simulink model "threephasethyristor"  (R2016a)
settings: Solver=VariableStepAuto  StartTime=0.0  StopTime=1  RelTol=1e-3
libraries: powerlib x21, powerlib_meascontrol x3, dspstat3 x1
settings Model: Creator=hakan  LastModifiedBy=hakan

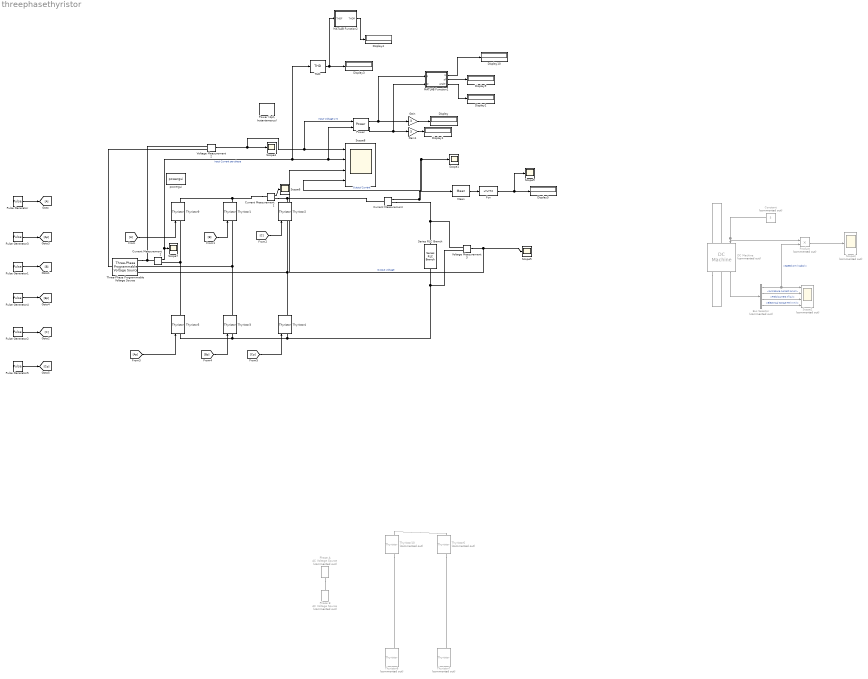
== system threephasethyristor ==
  Bus Selector : BusSelector  Commented=on  OutputSignals=Speed wm (rad/s),Armature current ia (A),Field current if (A),Electrical torque Te (n m)
  Constant : Constant  Commented=on  Value=5
  Current Measurement : powerlib/Measurements/Current Measurement  PhasorSimulation=off  OutputType=Complex  PSBequivalent=0
  Current Measurement1 : powerlib/Measurements/Current Measurement  PhasorSimulation=off  OutputType=Complex  PSBequivalent=0
  Current Measurement2 : powerlib/Measurements/Current Measurement  PhasorSimulation=off  OutputType=Complex  PSBequivalent=0
  DC Machine : powerlib/Machines/DC Machine  Commented=on  PresetModel=No  MechanicalLoad=Torque TL  FieldType=Wound  ShowDetailedParameters=on  MeasurementBus=off  RLa="[ 28  0.0133]"  RLf="[8260  6.4]"  Laf=1.5  MachineConstant=Torque constant (N.m/A)  Ke=1.8  Kt=1.8  J=1  Bm=0  Tf=0  w0=1  Ifinit=1  TsPowergui=0  TsBlock=-1
  Display{,1..5,9..10} (8 alike) : Display
  Fcn : Fcn  Expr=u*u*72
  Gain : Gain  Gain=3
  Gain1 : Gain  Gain=3
  MATLAB Function1 : MATLAB Function  TreatAsAtomicUnit=on
  MATLAB Function2 : MATLAB Function  TreatAsAtomicUnit=on
  Mean : dspstat3/Mean  run=off  reset_popup=None  InputProcessing=Columns as channels (frame based)  directionMode=Each column  dimension=1  roiEnable=off  roiType=Rectangles  roiPortion=Entire ROI  roiOutput=Individual statistics for each ROI  roiFlag=off  outputDataTypeStr=Inherit: Same as accumulator  outputLastDataTypeStr=Inherit: Same as accumulator  outputMin=[]  outputMax=[]  roundingMode=Floor  overflowMode=off
  Phase A : powerlib/Electrical Sources/AC Voltage Source  Commented=on  Amplitude=200  Phase=0  Frequency=50  SampleTime=0  Measurements=None  BusType=swing  Pref=10e3  Qref=0  Qmin=-inf  Qmax=+inf
  Phase B : powerlib/Electrical Sources/AC Voltage Source  Commented=on  Amplitude=200  Phase=120  Frequency=50  SampleTime=0  Measurements=None  BusType=swing  Pref=10e3  Qref=0  Qmin=-inf  Qmax=+inf
  Power : powerlib_meascontrol/Measurements/Power  Freq=50  Vinit=[1, 0]  Iinit=[1, 0]  Ts=0
  "Power (3ph, Instantaneous)" : powerlib_meascontrol/Measurements/Power (3ph, Instantaneous)
  Product : Product  Commented=on
  Pulse Generator : DiscretePulseGenerator  PulseType=Time based  Amplitude=2  Period=1/50  PulseWidth=5  PhaseDelay=(0/360)*20e-3+(30/360)*20e-3
  Pulse Generator1 : DiscretePulseGenerator  PulseType=Time based  Amplitude=2  Period=1/50  PulseWidth=5  PhaseDelay=(0/360)*20e-3+(120/360)*20e-3+(30/360)*20e-3
  Pulse Generator2 : DiscretePulseGenerator  PulseType=Time based  Amplitude=2  Period=1/50  PulseWidth=5  PhaseDelay=(0/360)*20e-3+(240/360)*20e-3+(30/360)*20e-3
  Pulse Generator3 : DiscretePulseGenerator  PulseType=Time based  Amplitude=2  Period=1/50  PulseWidth=5  PhaseDelay=(0/360)*20e-3+10e-3+(30/360)*20e-3
  Pulse Generator4 : DiscretePulseGenerator  PulseType=Time based  Amplitude=2  Period=1/50  PulseWidth=5  PhaseDelay=(0/360)*20e-3+10e-3+(120/360)*20e-3+(30/360)*20e-3
  Pulse Generator5 : DiscretePulseGenerator  PulseType=Time based  Amplitude=2  Period=1/50  PulseWidth=5  PhaseDelay=(0/360)*20e-3+10e-3+(240/360)*20e-3+(30/360)*20e-3
  Scope{1,4..7,9} (6 alike) : Scope
  Scope2 : Scope  Commented=on  NumInputPorts=4
  Scope3 : Scope  Commented=on
  Scope8 : Scope  NumInputPorts=4
  Series RLC Branch : powerlib/Elements/Series RLC Branch  LConnTagsString=__new0  RConnTagsString=__new0  BranchType=R  Resistance=72  Inductance=3*0.61/4  SetiL0=off  InitialCurrent=0  Capacitance=1e-6  Setx0=off  InitialVoltage=0  Measurements=None
  THD : powerlib_meascontrol/Measurements/THD  Freq=50  Ts=0
  Three-Phase Programmable Voltage Source : powerlib/Electrical Sources/Three-Phase Programmable Voltage Source  PositiveSequence=[245 0 50]  VariationEntity=None  VariationType=Table of time-amplitude pairs  VariationTypeAlt=Step  VariationStep=0.5  VariationRate=10  VariationMagnitude=0.3  VariationFrequency=2  VariationTiming=[1 2]  VariationPhaseA=off  Amplitudes=[1 0.8 1.2 1.0]  TimeValues=[0 0.1 0.15 0.2]  HarmonicGeneration=off  HarmonicA=[3 0.2 -25 0]  HarmonicB=[2 0.15 35 2]  Timing="[0.05  3]"  BusType=swing  Pref=0  Qref=0  Qmin=-inf  Qmax=inf
  Thyristor{1..5,9} (6 alike) : powerlib/Power Electronics/Thyristor  Ron=0.001  Lon=0  Vf=0.8  IC=0  Rs=500000  Cs=250e-9  Measurements=on
  Thyristor{6..8,10} (4 alike) : powerlib/Power Electronics/Thyristor  Commented=on  Ron=0.001  Lon=0  Vf=0.8  IC=0  Rs=500  Cs=250e-9  Measurements=on
  Voltage Measurement2 : powerlib/Measurements/Voltage Measurement  PhasorSimulation=off  OutputType=Complex  PSBequivalent=0
  Voltage Measurement3 : powerlib/Measurements/Voltage Measurement  PhasorSimulation=off  OutputType=Complex  PSBequivalent=0
  powergui : powerlib/powergui  Priority=1  SimulationMode=Discrete  SolverType=Tustin/Backward Euler (TBE)  SampleTime=50e-7*3  frequency=60  SPID=off  DisableSnubberDevices=off  DisableRonSwitches=off  DisableVfSwitches=off  SwTol=0  DisplayEquations=off  Interpol=off  ExternalGateDelay=off  methode=off  Ts=10  FunctionMessages=off  echomessages=off  HookPort=off  EnableUseOfTLC=off  x0status=blocks  frequencyindice=0  Pbase=100e6  ErrMax=1e-4  Iterations=50  UnitsV=kV  UnitsW=MW  buscounter=0  RestoreLinks=warning  ResistiveCurrentMeasurement=off  Frange=[0:2:500]  Ylog=off  Xlog=on  ShowGrid=off  save=off  variable=ZData  structure=0  ZoomFFT=off  StartTime=0.0  cycles=1  DisplayStyle=1  fundamental=60  FreqAxis=off  MaxFrequency=1000  frequencyindicesteady=1  RmsSteady=1  display=off
  wires:
  Pulse Generator1/1 -> [B]
  Pulse Generator2/1 -> [C]
  [A] -> Thyristor9/1
  [B] -> Thyristor1/1
  [C] -> Thyristor2/1
  [Ap] -> Thyristor5/1
  [Bp] -> Thyristor3/1
  [Cp] -> Thyristor4/1
  Pulse Generator/1 -> [A]
  Pulse Generator3/1 -> [Ap]
  Pulse Generator4/1 -> [Bp]
  Pulse Generator5/1 -> [Cp]
  DC Machine/1 -> Bus Selector/1
  Bus Selector/1 -> Product/2, Scope2/1  "<Speed wm (rad/s)>"
  Bus Selector/2 -> Scope2/2  "<Armature current ia (A)>"
  Bus Selector/3 -> Scope2/3  "<Field current if (A)>"
  Bus Selector/4 -> Scope2/4  "<Electrical torque Te (n m)>"
  Constant/1 -> Product/1, DC Machine/1
  Product/1 -> Scope3/1
  Current Measurement/1 -> Mean/1, Scope8/4, Scope1/1  "Output Current"
  Voltage Measurement2/1 -> Power/1, Scope8/1, Scope4/1  "Input Voltage L-N"
  Voltage Measurement3/1 -> Scope8/3, Scope5/1  "Output voltage"
  Current Measurement1/1 -> Scope6/1
  Current Measurement2/1 -> THD/1, Power/2, Scope8/2, Scope7/1  "Input Current per phase"
  Power/1 -> MATLAB Function1/1(P), Gain/1
  Power/2 -> MATLAB Function1/2(Q), Gain1/1
  MATLAB Function1/2(pf) -> Display9/1
  MATLAB Function1/1(S) -> Display10/1
  MATLAB Function1/3(angle) -> Display2/1
  THD/1 -> MATLAB Function2/1(THDF), Display3/1
  MATLAB Function2/1(THDR) -> Display4/1
  Fcn/1 -> Scope9/1, Display5/1
  Mean/1 -> Fcn/1
  Gain/1 -> Display/1
  Gain1/1 -> Display1/1
  connections:
  Phase A/LConn1 -- Phase B/LConn1
  Thyristor10/LConn1 -- Thyristor8/RConn1
  Thyristor10/RConn1 -- Thyristor6/RConn1
  Thyristor6/LConn1 -- Thyristor7/RConn1
  Thyristor4/LConn1 -- Voltage Measurement3/LConn2 -- Series RLC Branch/RConn1 -- Thyristor5/LConn1 -- Thyristor3/LConn1
  DC Machine/LConn2 -- DC Machine/LConn1
  Thyristor2/RConn1 -- Current Measurement/LConn1 -- Current Measurement1/RConn1
  DC Machine/RConn2 -- DC Machine/RConn1
  Current Measurement1/LConn1 -- Thyristor9/RConn1 -- Thyristor1/RConn1
  Current Measurement/RConn1 -- Voltage Measurement3/LConn1 -- Series RLC Branch/LConn1
  Voltage Measurement2/LConn2 -- Three-Phase Programmable Voltage Source/LConn1
  Voltage Measurement2/LConn1 -- Current Measurement2/LConn1 -- Three-Phase Programmable Voltage Source/RConn1
  Thyristor9/LConn1 -- Current Measurement2/RConn1 -- Thyristor5/RConn1
  Thyristor3/RConn1 -- Three-Phase Programmable Voltage Source/RConn2 -- Thyristor1/LConn1
  Thyristor4/RConn1 -- Three-Phase Programmable Voltage Source/RConn3 -- Thyristor2/LConn1

== matlab function threephasethyristor/MATLAB Function1 ==
  data: P input; S output; Q input; pf output; angle output
function [S,pf, angle] = fcn(P,Q)
S = sqrt(P^2 + Q^2);
pf = cos(atan(Q/P));
angle = (180/pi)*(atan(Q/P));

== matlab function threephasethyristor/MATLAB Function2 ==
  data: THDF input; THDR output
function THDR  = fcn(THDF)
THDR = THDF/(sqrt(1+THDF*THDF));
